simulink model "Leg_mech"  (R2015a)
settings: Solver=ode14x  StartTime=0.0  StopTime=inf  FixedStep=0.0006  RelTol=1e-3
values from neighbouring files (symbols this model uses):
  bL = 20.5    [prms.m]    (also in runFirst.m)
  bWb = 14.5    [prms.m]    (also in runFirst.m)
  bWs = 12.5    [prms.m]    (also in runFirst.m)
  C = CM + CL/n^2    (= 0.0001377500155)    [runFirst.m]
  d2 = 0    [prms.m]    (also in runFirst.m)
  J = JM + JL/n^2    (= 0.008455500031)    [runFirst.m]
  Ka = 12    [runFirst.m]
  Kb = 0.00867    [runFirst.m]
  Ke = 1    [runFirst.m]
  Km = 4.375    [runFirst.m]
  L = 0.0006    [runFirst.m]
  n = length(varargin)    [MyDynamixel.m]    (also in runFirst.m = 254)
  R = 1.4    [runFirst.m]
undefined symbols (not defined in the file or in its folder): X, Y, Z
undefined symbols (not defined in the file): L1, L2, L3, m1, m2, m3
libraries: sm_lib x20, nesl_utility x8
settings Model: Creator=340DANILOV  LastModifiedBy=340DANILOV
settings SolverCC: ZeroCrossAlgorithm=Adaptive
settings DataIOCC: SaveOutput=off  SaveTime=off
settings DiagnosticsConfigSet: SimMechanicsRigidlyBoundBlock=none

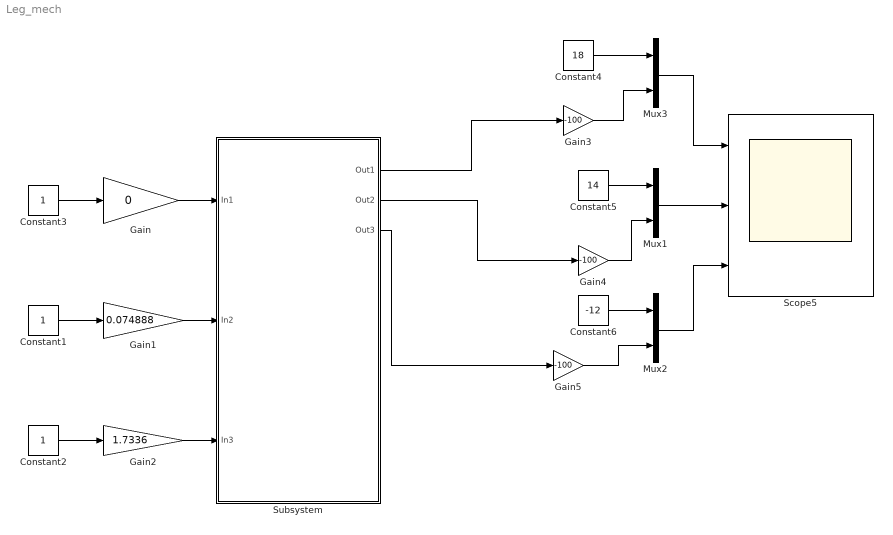
== system Leg_mech ==
  Constant1 : Constant
  Constant2 : Constant
  Constant3 : Constant
  Constant4 : Constant  Value=18
  Constant5 : Constant  Value=14
  Constant6 : Constant  Value=-12
  Gain : Gain  Gain=0
  Gain1 : Gain  Gain=0.074888
  Gain2 : Gain  Gain=1.7336
  Gain3 : Gain  Gain=-100
  Gain4 : Gain  Gain=-100
  Gain5 : Gain  Gain=-100
  Mux1 : Mux  Inputs=2
  Mux2 : Mux  Inputs=2
  Mux3 : Mux  Inputs=2
  Scope5 : Scope  NumInputPorts=3
      settings: YMin=14~14~-12.5  YMax=28~25~12.5  SaveName=ScopeData4
  Subsystem : Subsystem
  wires:
  Constant3/1 -> Gain/1
  Constant1/1 -> Gain1/1
  Constant2/1 -> Gain2/1
  Gain/1 -> Subsystem/1(In1)
  Gain1/1 -> Subsystem/2(In2)
  Gain2/1 -> Subsystem/3(In3)
  Mux2/1 -> Scope5/3
  Subsystem/1(Out1) -> Gain3/1
  Subsystem/2(Out2) -> Gain4/1
  Subsystem/3(Out3) -> Gain5/1
  Mux3/1 -> Scope5/1
  Mux1/1 -> Scope5/2
  Constant4/1 -> Mux3/1
  Gain3/1 -> Mux3/2
  Constant5/1 -> Mux1/1
  Gain4/1 -> Mux1/2
  Constant6/1 -> Mux2/1
  Gain5/1 -> Mux2/2

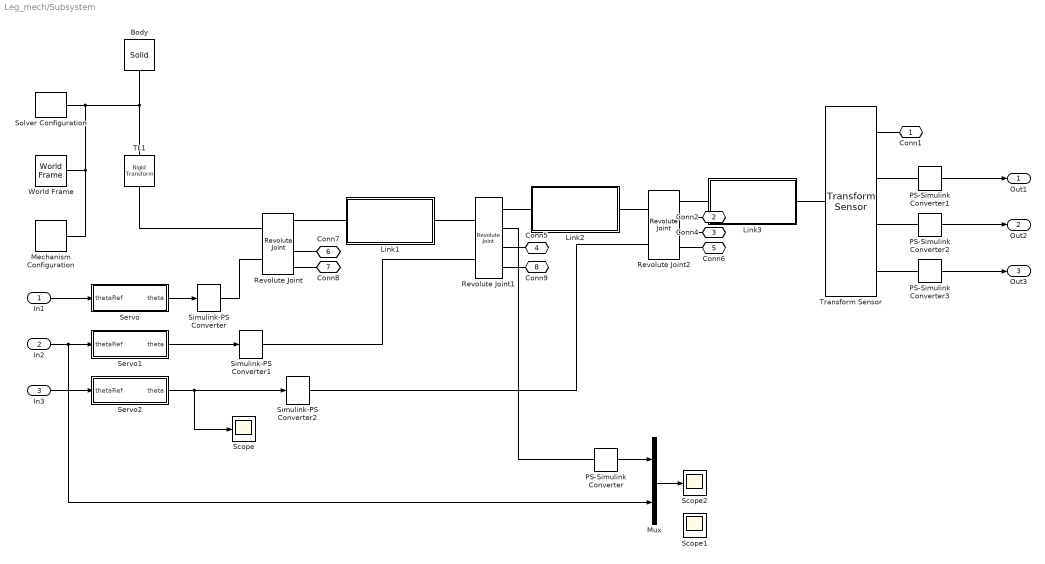
== system Leg_mech/Subsystem ==
  In1 : Inport
  In2 : Inport  Port=2
  In3 : Inport  Port=3
  Body : sm_lib/Body Elements/Solid  InertiaType=CalculateFromGeometry  Mass=0.835  MassUnits=kg  CenterOfMass=[0 0 0]  CenterOfMassUnits=m  MomentsOfInertia=[1 1 1]  MomentsOfInertiaUnits=kg*m^2  ProductsOfInertia=[0 0 0]  ProductsOfInertiaUnits=kg*m^2  DensityBased=off  Density=5000  DensityUnits=kg/(m^3)  GraphicType=FromGeometry  MarkerShape=Sphere  MarkerSize=10  MarkerSizeUnits=m  GraphicVisPropType=SimpleVisualProperties  GraphicDiffuseColor=[0.0 0.4 0.0]  GraphicSpecularColor=[0.5 0.5 0.5 1.0]  GraphicAmbientColor=[0.15 0.15 0.15 1.0]  GraphicEmissiveColor=[0.0 0.0 0.0 1.0]  GraphicShininess=75  GraphicOpacity=1.0  GeometryShape=GeneralExtrusion  RectangleSize=[1 1]  RectangleSizeUnits=m  BrickDimensions=[18.5 12.5 1]  BrickDimensionUnits=cm  CylinderRadius=1  CylinderRadiusUnits=m  CylinderLength=1  CylinderLengthUnits=m  SphereRadius=1  SphereRadiusUnits=m  EllipsoidRadii=[1 1 1]  EllipsoidRadiiUnits=m  ExtrusionCrossSection=[bL/2 bWs/2; 0 bWb/2; -bL/2 bWs/2; -bL/2 -bWs/2; 0 -bWb/2; bL/2 -bWs/2]  ExtrusionCrossSectionUnits=cm  ExtrusionLength=bH  ExtrusionLengthUnits=cm  PolygonNumSides=3  PolygonOuterRadius=1  PolygonOuterRadiusUnits=m  ExtGeomFileType=STEP  ExtGeomFileName=D:\Институт\Высертация\Model\3d\Body.STEP  ExtGeomFileUnits=m  RevolutionCrossSection=[1 1; 1 -1; 2 -1; 2 1]  RevolutionCrossSectionUnits=m  RevolutionExtent=Full  RevolutionAngle=180  RevolutionAngleUnits=deg  BlockFunction=simmechanics.library.body_elements.solid
  Link1 : Subsystem  mask{L=L1, W=1, H=1, m=m1, rgb=[0.1 0.1 0.90], Xangle=90, d1=-2.3}
      mask prompts: L "Length (cm)"; W "Width (cm)"; H "Thickness (cm)"; m "Mass (kg)"; rgb "Color [R G B]"; Xangle "+X Rotation (deg)"
      mask Display:
      | text(5,10, 'Link')
      | image(imread('sm_smpl_body.png'))
      | port_label('LConn',1,'L')
      | port_label('RConn',1,'R')
  Link2 : Subsystem  mask{L=L2, W=1, H=1, m=m2, rgb=[0.1 0.9 0.1], Xangle=180}
      mask prompts: L "Length (cm)"; W "Width (cm)"; H "Thickness (cm)"; m "Mass (kg)"; rgb "Color [R G B]"; Xangle "+X Rotation (deg)"
      mask Display:
      | text(5,10, 'Link')
      | image(imread('sm_smpl_body.png'))
      | port_label('LConn',1,'L')
      | port_label('RConn',1,'R')
  Link3 : Subsystem  mask{L=L3, W=1, H=1, m=m3, rgb=[0.9 0.1 0.10], Xangle=0}
      mask prompts: L "Length (cm)"; W "Width (cm)"; H "Thickness (cm)"; m "Mass (kg)"; rgb "Color [R G B]"; Xangle "+X Rotation (deg)"
      mask Display:
      | text(5,10, 'Link')
      | image(imread('sm_smpl_body.png'))
      | port_label('LConn',1,'L')
      | port_label('RConn',1,'R')
  Mechanism Configuration : sm_lib/Utilities/Mechanism Configuration  UniformGravity=Constant  GravityVector=[0 0 -9.80665]  GravityUnits=m/s^2  LinearizationDelta=0.001  BlockFunction=simmechanics.library.utilities.mechanism_configuration
  Mux : Mux  Inputs=2
  PS-Simulink Converter{,1..3} (4 alike) : nesl_utility/PS-Simulink Converter  PhysicalDomain=network_engine_domain  SubClassName=ps_output  LeftPortType=input  RightPortType=output  PseudoPeriodic=off  Frequencies=[]  Unit=1  AffineConversion=off
  Revolute Joint : sm_lib/Joints/Revolute Joint  SenseConstraintForce=off  SenseConstraintForceX=off  SenseConstraintForceY=off  SenseConstraintForceZ=off  SenseConstraintTorque=off  SenseConstraintTorqueX=off  SenseConstraintTorqueY=off  SenseConstraintTorqueZ=off  SenseTotalForce=off  SenseTotalForceX=off  SenseTotalForceY=off  SenseTotalForceZ=off  SenseTotalTorque=on  SenseTotalTorqueX=off  SenseTotalTorqueY=off  SenseTotalTorqueZ=off  CompositeWrenchDir=FollowerOnBase  CompositeWrenchFrame=BaseFrame  EquilibriumPosition=0  EquilibriumPositionUnits=deg  SpringStiffness=0  SpringStiffnessUnits=N*m/deg  DampingCoefficient=0  DampingCoefficientUnits=N*m/(deg/s)  TorqueActuationMode=ComputedTorque  MotionActuationMode=InputMotion  SensePosition=on  SenseVelocity=off  SenseAcceleration=off  SenseTorqueForce=on  PositionTargetSpecify=off  PositionTargetPriority=High  PositionTargetValue=0  PositionTargetValueUnits=deg  VelocityTargetSpecify=off  VelocityTargetPriority=High  VelocityTargetValue=0  VelocityTargetValueUnits=deg/s  BlockFunction=simmechanics.library.joints.revolute_joint
  Revolute Joint1 : sm_lib/Joints/Revolute Joint  SenseConstraintForce=off  SenseConstraintForceX=off  SenseConstraintForceY=off  SenseConstraintForceZ=off  SenseConstraintTorque=off  SenseConstraintTorqueX=off  SenseConstraintTorqueY=off  SenseConstraintTorqueZ=off  SenseTotalForce=off  SenseTotalForceX=off  SenseTotalForceY=off  SenseTotalForceZ=off  SenseTotalTorque=on  SenseTotalTorqueX=off  SenseTotalTorqueY=off  SenseTotalTorqueZ=off  CompositeWrenchDir=FollowerOnBase  CompositeWrenchFrame=BaseFrame  EquilibriumPosition=0  EquilibriumPositionUnits=deg  SpringStiffness=0  SpringStiffnessUnits=N*m/deg  DampingCoefficient=0  DampingCoefficientUnits=N*m/(deg/s)  TorqueActuationMode=ComputedTorque  MotionActuationMode=InputMotion  SensePosition=on  SenseVelocity=off  SenseAcceleration=off  SenseTorqueForce=on  PositionTargetSpecify=off  PositionTargetPriority=High  PositionTargetValue=0  PositionTargetValueUnits=deg  VelocityTargetSpecify=off  VelocityTargetPriority=High  VelocityTargetValue=0  VelocityTargetValueUnits=deg/s  BlockFunction=simmechanics.library.joints.revolute_joint
  Revolute Joint2 : sm_lib/Joints/Revolute Joint  SenseConstraintForce=off  SenseConstraintForceX=off  SenseConstraintForceY=off  SenseConstraintForceZ=off  SenseConstraintTorque=off  SenseConstraintTorqueX=off  SenseConstraintTorqueY=off  SenseConstraintTorqueZ=off  SenseTotalForce=off  SenseTotalForceX=off  SenseTotalForceY=off  SenseTotalForceZ=off  SenseTotalTorque=on  SenseTotalTorqueX=off  SenseTotalTorqueY=off  SenseTotalTorqueZ=off  CompositeWrenchDir=FollowerOnBase  CompositeWrenchFrame=BaseFrame  EquilibriumPosition=0  EquilibriumPositionUnits=deg  SpringStiffness=0  SpringStiffnessUnits=N*m/deg  DampingCoefficient=0  DampingCoefficientUnits=N*m/(deg/s)  TorqueActuationMode=ComputedTorque  MotionActuationMode=InputMotion  SensePosition=on  SenseVelocity=off  SenseAcceleration=off  SenseTorqueForce=on  PositionTargetSpecify=off  PositionTargetPriority=High  PositionTargetValue=0  PositionTargetValueUnits=deg  VelocityTargetSpecify=off  VelocityTargetPriority=High  VelocityTargetValue=0  VelocityTargetValueUnits=deg/s  BlockFunction=simmechanics.library.joints.revolute_joint
  Scope : Scope
  Scope1 : Scope
  Scope2 : Scope
      settings: YMin=0.025  YMax=0.3  SaveName=ScopeData2
  Servo : Subsystem
  Servo1 : Subsystem
  Servo2 : Subsystem
  Simulink-PS Converter : nesl_utility/Simulink-PS Converter  PhysicalDomain=network_engine_domain  SubClassName=ps_input  LeftPortType=input  RightPortType=output  PseudoPeriodic=off  Frequencies=[]  NoiseDistribution=none  NoiseParameters=[]  Unit=1  AffineConversion=off  InputFiltering=on  SimscapeFilterOrder=2  InputFilterTimeConstant=0.001  UdotUserProvided=1
  Simulink-PS Converter1 : nesl_utility/Simulink-PS Converter  PhysicalDomain=network_engine_domain  SubClassName=ps_input  LeftPortType=input  RightPortType=output  PseudoPeriodic=off  Frequencies=[]  NoiseDistribution=none  NoiseParameters=[]  Unit=1  AffineConversion=off  InputFiltering=on  SimscapeFilterOrder=2  InputFilterTimeConstant=0.001  UdotUserProvided=1
  Simulink-PS Converter2 : nesl_utility/Simulink-PS Converter  PhysicalDomain=network_engine_domain  SubClassName=ps_input  LeftPortType=input  RightPortType=output  PseudoPeriodic=off  Frequencies=[]  NoiseDistribution=none  NoiseParameters=[]  Unit=1  AffineConversion=off  InputFiltering=on  SimscapeFilterOrder=2  InputFilterTimeConstant=0.001  UdotUserProvided=1
  Solver Configuration : nesl_utility/Solver Configuration  PhysicalDomain=network_engine_domain  SubClassName=solver  LeftPortType=input  RightPortType=generic  Accelerate=off  Tones=[]  Harmonics=[]  SimulateNoise=off  Profile=off  UseLocalSampling=off  EnableSwitchedLinearOptims=on  FrequencyDomain=off  UseCCode=off  RelTol=0.001  AbsTol=1e-06  MinStep=1e-09  ToWorkspace=off  RevertToSquareIcSolve=off  NumHomotopyIterations=100  DoDC=off  ResidualTolerance=1e-09  UseLocalSolver=off  LocalSolverChoice=NE_BACKWARD_EULER_ADVANCER  LocalSolverSampleTime=0.001  DoFixedCost=off  MaxNonlinIter=3  MaxModeIter=2  LinearAlgebra=Sparse  DelaysMemoryBudget=1024  AutomaticFiltering=on  FilteringTimeConstant=0.001
  TL1 : sm_lib/Frames and Transforms/Rigid Transform  TranslationMethod=Cartesian  TranslationLengthUnit=cm  TranslationStandardAxis=+Z  TranslationStandardOffset=0  TranslationCartesianOffset=[bL/2 bWs/2 0]  TranslationROffset=0  TranslationROffsetUnits=m  TranslationZOffset=0  TranslationZOffsetUnits=m  TranslationThetaOffset=0  TranslationThetaOffsetUnits=deg  RotationMethod=StandardAxis  RotationAngleUnits=deg  RotationStandardAxis=+Z  RotationAngle=90-45  RotationArbitraryAxis=[0 0 1]  FollAlignAxisA=+X  BaseAlignAxisA=+Y  FollAlignAxisB=+Y  BaseAlignAxisB=+Z  RotationMatrix=[1 0 0; 0 1 0; 0 0 1]  BlockFunction=simmechanics.library.frames_transforms.rigid_transform
  Transform Sensor : sm_lib/Frames and Transforms/Transform Sensor  MeasurementFrame=World  SenseAngle=off  SenseAxis=off  SenseAngle1=off  SenseAngle2=off  SenseAngle3=off  SenseQ=off  SenseR=off  SenseOmegaX=off  SenseOmegaY=off  SenseOmegaZ=off  SenseOmega1=off  SenseOmega2=off  SenseOmega3=off  SenseQDot=off  SenseRDot=off  SenseAlphaX=off  SenseAlphaY=off  SenseAlphaZ=off  SenseAlpha1=off  SenseAlpha2=off  SenseAlpha3=off  SenseQDDot=off  SenseRDDot=off  SenseX=on  SenseY=on  SenseZ=on  SenseRad=off  SenseAzim=off  SenseDist=off  SenseInc=off  SenseXDot=off  SenseYDot=off  SenseZDot=off  SenseRadDot=off  SenseAzimDot=off  SenseDistDot=off  SenseIncDot=off  SenseXDDot=off  SenseYDDot=off  SenseZDDot=off  SenseRadDDot=off  SenseAzimDDot=off  SenseDistDDot=off  SenseIncDDot=off  BlockFunction=simmechanics.library.frames_transforms.transform_sensor
  World Frame : sm_lib/Frames and Transforms/World Frame  BlockFunction=simmechanics.library.frames_transforms.world_frame
  Conn1 : PMIOPort  Port=1  Side=Right
  Conn2 : PMIOPort  Port=2  Side=Right
  Conn4 : PMIOPort  Port=3  Side=Right
  Conn5 : PMIOPort  Port=4  Side=Right
  Conn6 : PMIOPort  Port=5  Side=Right
  Conn7 : PMIOPort  Port=6  Side=Right
  Conn8 : PMIOPort  Port=7  Side=Right
  Conn9 : PMIOPort  Port=8  Side=Right
  Out1 : Outport
  Out2 : Outport  Port=2
  Out3 : Outport  Port=3
  wires:
  PS-Simulink Converter2/1 -> Out2/1
  PS-Simulink Converter1/1 -> Out1/1
  Servo/1(theta) -> Simulink-PS Converter/1
  Servo2/1(theta) -> Scope/1, Simulink-PS Converter2/1
  Servo1/1(theta) -> Simulink-PS Converter1/1
  In1/1 -> Servo/1(thetaRef)
  In2/1 -> Mux/2, Servo1/1(thetaRef)
  In3/1 -> Servo2/1(thetaRef)
  PS-Simulink Converter3/1 -> Out3/1
  PS-Simulink Converter/1 -> Mux/1
  Mux/1 -> Scope2/1
  connections:
  PS-Simulink Converter1/LConn1 -- Transform Sensor/RConn2
  World Frame/RConn1 -- Mechanism Configuration/RConn1 -- Body/RConn1 -- TL1/LConn1 -- Solver Configuration/RConn1
  Revolute Joint/LConn1 -- TL1/RConn1
  Link1/LConn1 -- Revolute Joint/RConn1
  Revolute Joint1/LConn1 -- Link1/RConn1
  Link2/LConn1 -- Revolute Joint1/RConn1
  Revolute Joint2/LConn1 -- Link2/RConn1
  Link3/LConn1 -- Revolute Joint2/RConn1
  Revolute Joint/LConn2 -- Simulink-PS Converter/RConn1
  Simulink-PS Converter1/RConn1 -- Revolute Joint1/LConn2
  Simulink-PS Converter2/RConn1 -- Revolute Joint2/LConn2
  Transform Sensor/RConn1 -- Conn1/RConn1
  Revolute Joint/RConn4 -- Conn8/RConn1
  Revolute Joint1/RConn3 -- Conn5/RConn1
  Revolute Joint1/RConn4 -- Conn9/RConn1
  Revolute Joint2/RConn4 -- Conn6/RConn1
  Revolute Joint2/RConn3 -- Conn4/RConn1
  PS-Simulink Converter/LConn1 -- Revolute Joint1/RConn2
  Revolute Joint2/RConn2 -- Conn2/RConn1
  Revolute Joint/RConn3 -- Conn7/RConn1
  PS-Simulink Converter2/LConn1 -- Transform Sensor/RConn3
  Transform Sensor/LConn1 -- Link3/RConn1
  PS-Simulink Converter3/LConn1 -- Transform Sensor/RConn4

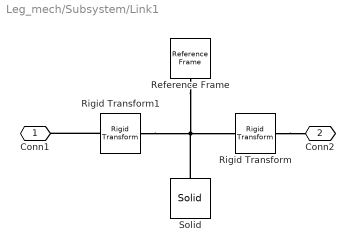
== system Leg_mech/Subsystem/Link1 ==
  Reference Frame : sm_lib/Frames and Transforms/Reference Frame  BlockFunction=simmechanics.library.frames_transforms.reference_frame
  Rigid Transform : sm_lib/Frames and Transforms/Rigid Transform  TranslationMethod=Cartesian  TranslationLengthUnit=cm  TranslationStandardAxis=+X  TranslationStandardOffset=L/2  TranslationCartesianOffset=[L/2 0 d2]  TranslationROffset=0  TranslationROffsetUnits=m  TranslationZOffset=0  TranslationZOffsetUnits=m  TranslationThetaOffset=0  TranslationThetaOffsetUnits=deg  RotationMethod=StandardAxis  RotationAngleUnits=deg  RotationStandardAxis=+X  RotationAngle=Xangle  RotationArbitraryAxis=[0 0 1]  FollAlignAxisA=+X  BaseAlignAxisA=+Y  FollAlignAxisB=+Y  BaseAlignAxisB=+Z  RotationMatrix=[1 0 0; 0 1 0; 0 0 1]  BlockFunction=simmechanics.library.frames_transforms.rigid_transform
  Rigid Transform1 : sm_lib/Frames and Transforms/Rigid Transform  TranslationMethod=StandardAxis  TranslationLengthUnit=cm  TranslationStandardAxis=-X  TranslationStandardOffset=L/2  TranslationCartesianOffset=[0 0 0]  TranslationROffset=0  TranslationROffsetUnits=m  TranslationZOffset=0  TranslationZOffsetUnits=m  TranslationThetaOffset=0  TranslationThetaOffsetUnits=deg  RotationMethod=None  RotationAngleUnits=deg  RotationStandardAxis=+Z  RotationAngle=0.0  RotationArbitraryAxis=[0 0 1]  FollAlignAxisA=+X  BaseAlignAxisA=+Y  FollAlignAxisB=+Y  BaseAlignAxisB=+Z  RotationMatrix=[1 0 0; 0 1 0; 0 0 1]  BlockFunction=simmechanics.library.frames_transforms.rigid_transform
  Solid : sm_lib/Body Elements/Solid  InertiaType=PointMass  Mass=m  MassUnits=kg  CenterOfMass=[0 0 0]  CenterOfMassUnits=m  MomentsOfInertia=[1 1 1]  MomentsOfInertiaUnits=kg*m^2  ProductsOfInertia=[0 0 0]  ProductsOfInertiaUnits=kg*m^2  DensityBased=off  Density=1  DensityUnits=kg/(m^3)  GraphicType=FromGeometry  MarkerShape=Sphere  MarkerSize=10  MarkerSizeUnits=m  GraphicVisPropType=SimpleVisualProperties  GraphicDiffuseColor=rgb  GraphicSpecularColor=[0.5 0.5 0.5 1.0]  GraphicAmbientColor=[0.15 0.15 0.15 1.0]  GraphicEmissiveColor=[0.0 0.0 0.0 1.0]  GraphicShininess=75  GraphicOpacity=1.0  GeometryShape=Brick  RectangleSize=[1 1]  RectangleSizeUnits=m  BrickDimensions=[L 1 1]  BrickDimensionUnits=cm  CylinderRadius=1  CylinderRadiusUnits=m  CylinderLength=1  CylinderLengthUnits=m  SphereRadius=1  SphereRadiusUnits=m  EllipsoidRadii=[1 1 1]  EllipsoidRadiiUnits=m  ExtrusionCrossSection=[1 1; -1 1; -1 -1; 1 -1]  ExtrusionCrossSectionUnits=m  ExtrusionLength=1  ExtrusionLengthUnits=m  PolygonNumSides=3  PolygonOuterRadius=1  PolygonOuterRadiusUnits=m  ExtGeomFileType=STEP  ExtGeomFileName=D:\Институт\Высертация\Model\3d\Link1.STEP  ExtGeomFileUnits=m  RevolutionCrossSection=[1 1; 1 -1; 2 -1; 2 1]  RevolutionCrossSectionUnits=m  RevolutionExtent=Full  RevolutionAngle=180  RevolutionAngleUnits=deg  BlockFunction=simmechanics.library.body_elements.solid
  Conn1 : PMIOPort  Port=1  Side=Left
  Conn2 : PMIOPort  Port=2  Side=Right
  connections:
  Reference Frame/RConn1 -- Solid/RConn1 -- Rigid Transform/LConn1 -- Rigid Transform1/LConn1
  Rigid Transform/RConn1 -- Conn2/RConn1
  Rigid Transform1/RConn1 -- Conn1/RConn1

== system Leg_mech/Subsystem/Link2 ==
  Reference Frame : sm_lib/Frames and Transforms/Reference Frame  BlockFunction=simmechanics.library.frames_transforms.reference_frame
  Rigid Transform : sm_lib/Frames and Transforms/Rigid Transform  TranslationMethod=StandardAxis  TranslationLengthUnit=cm  TranslationStandardAxis=+X  TranslationStandardOffset=L/2  TranslationCartesianOffset=[0 0 0]  TranslationROffset=0  TranslationROffsetUnits=m  TranslationZOffset=0  TranslationZOffsetUnits=m  TranslationThetaOffset=0  TranslationThetaOffsetUnits=deg  RotationMethod=StandardAxis  RotationAngleUnits=deg  RotationStandardAxis=+X  RotationAngle=Xangle  RotationArbitraryAxis=[0 0 1]  FollAlignAxisA=+X  BaseAlignAxisA=+Y  FollAlignAxisB=+Y  BaseAlignAxisB=+Z  RotationMatrix=[1 0 0; 0 1 0; 0 0 1]  BlockFunction=simmechanics.library.frames_transforms.rigid_transform
  Rigid Transform1 : sm_lib/Frames and Transforms/Rigid Transform  TranslationMethod=StandardAxis  TranslationLengthUnit=cm  TranslationStandardAxis=-X  TranslationStandardOffset=L/2  TranslationCartesianOffset=[0 0 0]  TranslationROffset=0  TranslationROffsetUnits=m  TranslationZOffset=0  TranslationZOffsetUnits=m  TranslationThetaOffset=0  TranslationThetaOffsetUnits=deg  RotationMethod=None  RotationAngleUnits=deg  RotationStandardAxis=+Z  RotationAngle=0.0  RotationArbitraryAxis=[0 0 1]  FollAlignAxisA=+X  BaseAlignAxisA=+Y  FollAlignAxisB=+Y  BaseAlignAxisB=+Z  RotationMatrix=[1 0 0; 0 1 0; 0 0 1]  BlockFunction=simmechanics.library.frames_transforms.rigid_transform
  Solid : sm_lib/Body Elements/Solid  InertiaType=PointMass  Mass=m  MassUnits=kg  CenterOfMass=[0 0 0]  CenterOfMassUnits=m  MomentsOfInertia=[1 1 1]  MomentsOfInertiaUnits=kg*m^2  ProductsOfInertia=[0 0 0]  ProductsOfInertiaUnits=kg*m^2  DensityBased=off  Density=1  DensityUnits=kg/(m^3)  GraphicType=FromGeometry  MarkerShape=Sphere  MarkerSize=10  MarkerSizeUnits=m  GraphicVisPropType=SimpleVisualProperties  GraphicDiffuseColor=rgb  GraphicSpecularColor=[0.5 0.5 0.5 1.0]  GraphicAmbientColor=[0.15 0.15 0.15 1.0]  GraphicEmissiveColor=[0.0 0.0 0.0 1.0]  GraphicShininess=75  GraphicOpacity=1.0  GeometryShape=Brick  RectangleSize=[1 1]  RectangleSizeUnits=m  BrickDimensions=[L W H]  BrickDimensionUnits=cm  CylinderRadius=1  CylinderRadiusUnits=m  CylinderLength=1  CylinderLengthUnits=m  SphereRadius=1  SphereRadiusUnits=m  EllipsoidRadii=[1 1 1]  EllipsoidRadiiUnits=m  ExtrusionCrossSection=[1 1; -1 1; -1 -1; 1 -1]  ExtrusionCrossSectionUnits=m  ExtrusionLength=1  ExtrusionLengthUnits=m  PolygonNumSides=3  PolygonOuterRadius=1  PolygonOuterRadiusUnits=m  ExtGeomFileType=STEP  ExtGeomFileName=D:\Институт\Высертация\Model\3d\Link2.STEP  ExtGeomFileUnits=m  RevolutionCrossSection=[1 1; 1 -1; 2 -1; 2 1]  RevolutionCrossSectionUnits=m  RevolutionExtent=Full  RevolutionAngle=180  RevolutionAngleUnits=deg  BlockFunction=simmechanics.library.body_elements.solid
  Conn1 : PMIOPort  Port=1  Side=Left
  Conn2 : PMIOPort  Port=2  Side=Right
  connections:
  Rigid Transform1/RConn1 -- Conn1/RConn1
  Rigid Transform/RConn1 -- Conn2/RConn1
  Rigid Transform1/LConn1 -- Rigid Transform/LConn1 -- Solid/RConn1 -- Reference Frame/RConn1

== system Leg_mech/Subsystem/Link3 ==
  Reference Frame : sm_lib/Frames and Transforms/Reference Frame  BlockFunction=simmechanics.library.frames_transforms.reference_frame
  Rigid Transform : sm_lib/Frames and Transforms/Rigid Transform  TranslationMethod=StandardAxis  TranslationLengthUnit=cm  TranslationStandardAxis=+X  TranslationStandardOffset=L/2  TranslationCartesianOffset=[0 0 0]  TranslationROffset=0  TranslationROffsetUnits=m  TranslationZOffset=0  TranslationZOffsetUnits=m  TranslationThetaOffset=0  TranslationThetaOffsetUnits=deg  RotationMethod=None  RotationAngleUnits=deg  RotationStandardAxis=+X  RotationAngle=Xangle  RotationArbitraryAxis=[0 0 1]  FollAlignAxisA=+X  BaseAlignAxisA=+Y  FollAlignAxisB=+Y  BaseAlignAxisB=+Z  RotationMatrix=[1 0 0; 0 1 0; 0 0 1]  BlockFunction=simmechanics.library.frames_transforms.rigid_transform
  Rigid Transform1 : sm_lib/Frames and Transforms/Rigid Transform  TranslationMethod=StandardAxis  TranslationLengthUnit=cm  TranslationStandardAxis=-X  TranslationStandardOffset=L/2  TranslationCartesianOffset=[0 0 0]  TranslationROffset=0  TranslationROffsetUnits=m  TranslationZOffset=0  TranslationZOffsetUnits=m  TranslationThetaOffset=0  TranslationThetaOffsetUnits=deg  RotationMethod=None  RotationAngleUnits=deg  RotationStandardAxis=+Z  RotationAngle=0.0  RotationArbitraryAxis=[0 0 1]  FollAlignAxisA=+X  BaseAlignAxisA=+Y  FollAlignAxisB=+Y  BaseAlignAxisB=+Z  RotationMatrix=[1 0 0; 0 1 0; 0 0 1]  BlockFunction=simmechanics.library.frames_transforms.rigid_transform
  Solid : sm_lib/Body Elements/Solid  InertiaType=PointMass  Mass=m  MassUnits=kg  CenterOfMass=[0 0 0]  CenterOfMassUnits=m  MomentsOfInertia=[1 1 1]  MomentsOfInertiaUnits=kg*m^2  ProductsOfInertia=[0 0 0]  ProductsOfInertiaUnits=kg*m^2  DensityBased=off  Density=1  DensityUnits=kg/(m^3)  GraphicType=FromGeometry  MarkerShape=Sphere  MarkerSize=10  MarkerSizeUnits=m  GraphicVisPropType=SimpleVisualProperties  GraphicDiffuseColor=rgb  GraphicSpecularColor=[0.5 0.5 0.5 1.0]  GraphicAmbientColor=[0.15 0.15 0.15 1.0]  GraphicEmissiveColor=[0.0 0.0 0.0 1.0]  GraphicShininess=75  GraphicOpacity=1.0  GeometryShape=Brick  RectangleSize=[1 1]  RectangleSizeUnits=m  BrickDimensions=[L W H]  BrickDimensionUnits=cm  CylinderRadius=1  CylinderRadiusUnits=m  CylinderLength=1  CylinderLengthUnits=m  SphereRadius=1  SphereRadiusUnits=m  EllipsoidRadii=[1 1 1]  EllipsoidRadiiUnits=m  ExtrusionCrossSection=[1 1; -1 1; -1 -1; 1 -1]  ExtrusionCrossSectionUnits=m  ExtrusionLength=1  ExtrusionLengthUnits=m  PolygonNumSides=3  PolygonOuterRadius=1  PolygonOuterRadiusUnits=m  ExtGeomFileType=STEP  ExtGeomFileName=D:\Институт\Высертация\Model\3d\link3.STEP  ExtGeomFileUnits=m  RevolutionCrossSection=[1 1; 1 -1; 2 -1; 2 1]  RevolutionCrossSectionUnits=m  RevolutionExtent=Full  RevolutionAngle=180  RevolutionAngleUnits=deg  BlockFunction=simmechanics.library.body_elements.solid
  Conn1 : PMIOPort  Port=1  Side=Left
  Conn2 : PMIOPort  Port=2  Side=Right
  connections:
  Reference Frame/RConn1 -- Solid/RConn1 -- Rigid Transform/LConn1 -- Rigid Transform1/LConn1
  Rigid Transform/RConn1 -- Conn2/RConn1
  Rigid Transform1/RConn1 -- Conn1/RConn1

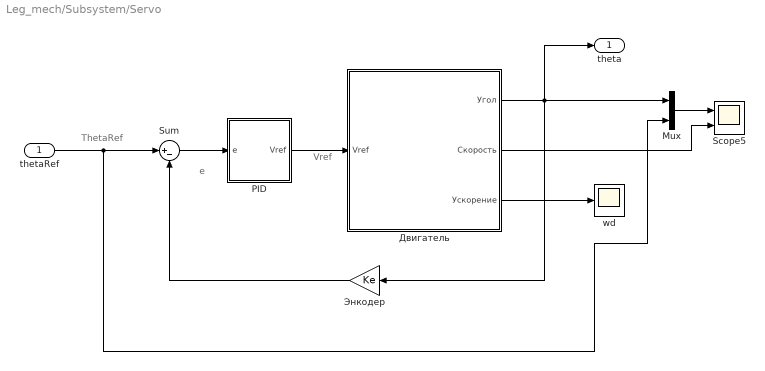
== system Leg_mech/Subsystem/Servo ==
  note: ThetaRef
  note: e
  note: Vref
  thetaRef : Inport
  Mux : Mux  Inputs=2
  PID : Subsystem
  Scope5 : Scope  NumInputPorts=2
      settings: YMin=5.55112e-17~-3.5  YMax=1.1~3.5  SaveName=ScopeData45
  Sum : Sum  Inputs=|+-
  wd : Scope
      settings: SaveName=ScopeData3
  Двигатель : Subsystem
  Энкодер : Gain  Gain=Ke
  theta : Outport
  wires:
  Mux/1 -> Scope5/1
  Двигатель/3(Ускорение) -> wd/1
  PID/1(Vref) -> Двигатель/1(Vref)
  Двигатель/1(Угол) -> Энкодер/1, theta/1, Mux/1
  Энкодер/1 -> Sum/2
  Sum/1 -> PID/1(e)
  thetaRef/1 -> Sum/1, Mux/2
  Двигатель/2(Скорость) -> Scope5/2

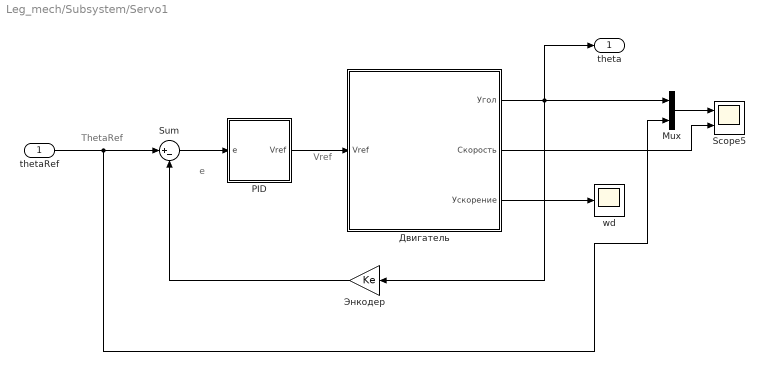
== system Leg_mech/Subsystem/Servo1 ==
  note: ThetaRef
  note: e
  note: Vref
  thetaRef : Inport
  Mux : Mux  Inputs=2
  PID : Subsystem
  Scope5 : Scope  NumInputPorts=2
      settings: YMin=-0.28285~-0.0045  YMax=-0.2824~0  SaveName=ScopeData45
  Sum : Sum  Inputs=|+-
  wd : Scope
      settings: SaveName=ScopeData3
  Двигатель : Subsystem
  Энкодер : Gain  Gain=Ke
  theta : Outport
  wires:
  Mux/1 -> Scope5/1
  Двигатель/3(Ускорение) -> wd/1
  PID/1(Vref) -> Двигатель/1(Vref)
  Двигатель/1(Угол) -> Энкодер/1, theta/1, Mux/1
  Энкодер/1 -> Sum/2
  Sum/1 -> PID/1(e)
  thetaRef/1 -> Sum/1, Mux/2
  Двигатель/2(Скорость) -> Scope5/2

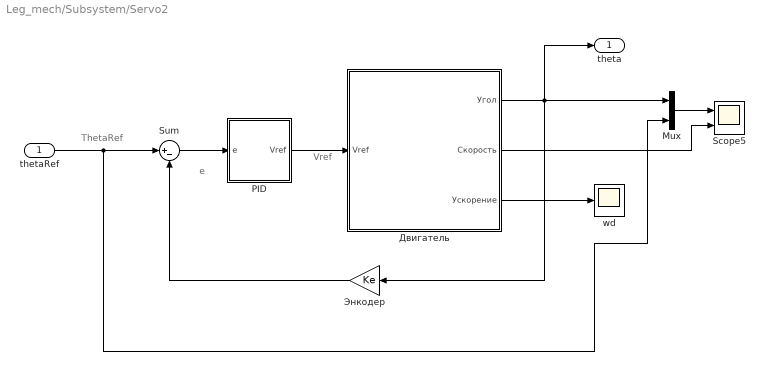
== system Leg_mech/Subsystem/Servo2 ==
  note: Vref
  note: e
  note: ThetaRef
  thetaRef : Inport
  Mux : Mux  Inputs=2
  PID : Subsystem
  Scope5 : Scope  NumInputPorts=2
      settings: YMin=1.4~-0.25  YMax=2.2~3.25  SaveName=ScopeData45
  Sum : Sum  Inputs=|+-
  wd : Scope
      settings: SaveName=ScopeData3
  Двигатель : Subsystem
  Энкодер : Gain  Gain=Ke
  theta : Outport
  wires:
  Двигатель/2(Скорость) -> Scope5/2
  thetaRef/1 -> Mux/2, Sum/1
  Sum/1 -> PID/1(e)
  Энкодер/1 -> Sum/2
  Двигатель/1(Угол) -> Mux/1, theta/1, Энкодер/1
  PID/1(Vref) -> Двигатель/1(Vref)
  Двигатель/3(Ускорение) -> wd/1
  Mux/1 -> Scope5/1

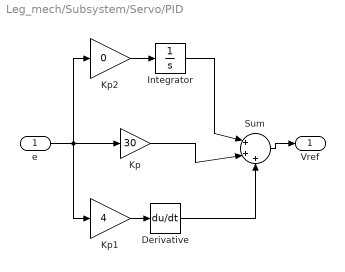
== system Leg_mech/Subsystem/Servo/PID ==
  e : Inport
  Derivative : Derivative
  Integrator : Integrator
  Kp : Gain  Gain=30
  Kp1 : Gain  Gain=4
  Kp2 : Gain  Gain=0
  Sum : Sum  Inputs=|+++
  Vref : Outport
  wires:
  Derivative/1 -> Sum/3
  Kp/1 -> Sum/2
  Integrator/1 -> Sum/1
  Kp2/1 -> Integrator/1
  Sum/1 -> Vref/1
  Kp1/1 -> Derivative/1
  e/1 -> Kp/1, Kp1/1, Kp2/1

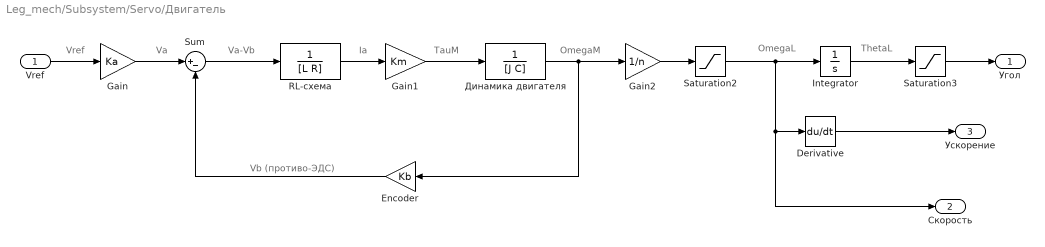
== system Leg_mech/Subsystem/Servo/Двигатель ==
  note: Vref
  note: Va
  note: Va-Vb
  note: Vb (противо-ЭДС)
  note: Ia
  note: TauM
  note: OmegaM
  note: OmegaL
  note: ThetaL
  Vref : Inport
  Derivative : Derivative
  Encoder : Gain  Gain=Kb
  Gain : Gain  Gain=Ka
  Gain1 : Gain  Gain=Km
  Gain2 : Gain  Gain=1/n
  Integrator : Integrator
  RL-схема : TransferFcn  Denominator=[L R]
  Saturation2 : Saturate  UpperLimit=190*pi/180  LowerLimit=-190*pi/180  OutMin=[-190*pi/180]  OutMax=[190*pi/180]
  Saturation3 : Saturate  UpperLimit=60*pi/180  LowerLimit=-60*pi/180  OutMin=[-150*pi/180]  OutMax=[150*pi/180]
  Sum : Sum  Inputs=|+-
  Динамика двигателя : TransferFcn  Denominator=[J C]
  Угол : Outport
  Скорость : Outport  Port=2
  Ускорение : Outport  Port=3
  wires:
  Saturation3/1 -> Угол/1
  Gain/1 -> Sum/1
  Vref/1 -> Gain/1
  Integrator/1 -> Saturation3/1
  Encoder/1 -> Sum/2
  Gain1/1 -> Динамика двигателя/1
  Sum/1 -> RL-схема/1
  RL-схема/1 -> Gain1/1
  Derivative/1 -> Ускорение/1
  Динамика двигателя/1 -> Gain2/1, Encoder/1
  Gain2/1 -> Saturation2/1
  Saturation2/1 -> Integrator/1, Скорость/1, Derivative/1

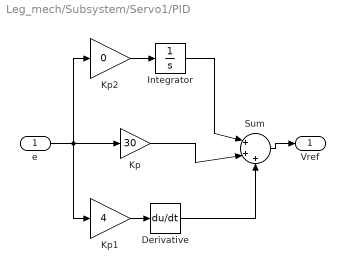
== system Leg_mech/Subsystem/Servo1/PID ==
  e : Inport
  Derivative : Derivative
  Integrator : Integrator
  Kp : Gain  Gain=30
  Kp1 : Gain  Gain=4
  Kp2 : Gain  Gain=0
  Sum : Sum  Inputs=|+++
  Vref : Outport
  wires:
  Derivative/1 -> Sum/3
  Kp/1 -> Sum/2
  Integrator/1 -> Sum/1
  Kp2/1 -> Integrator/1
  Sum/1 -> Vref/1
  Kp1/1 -> Derivative/1
  e/1 -> Kp/1, Kp1/1, Kp2/1

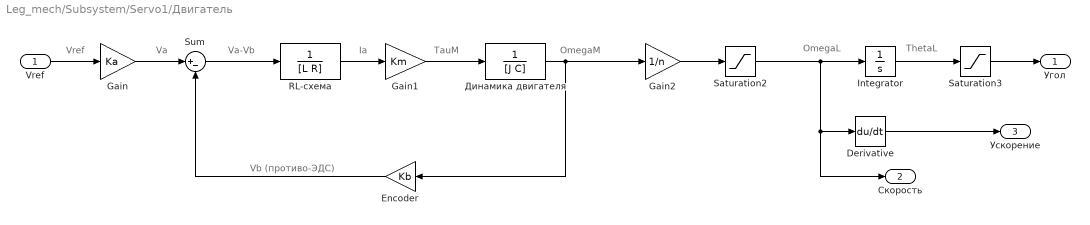
== system Leg_mech/Subsystem/Servo1/Двигатель ==
  note: Vref
  note: Va
  note: Va-Vb
  note: Vb (противо-ЭДС)
  note: Ia
  note: TauM
  note: OmegaM
  note: OmegaL
  note: ThetaL
  Vref : Inport
  Derivative : Derivative
  Encoder : Gain  Gain=Kb
  Gain : Gain  Gain=Ka
  Gain1 : Gain  Gain=Km
  Gain2 : Gain  Gain=1/n
  Integrator : Integrator
  RL-схема : TransferFcn  Denominator=[L R]
  Saturation2 : Saturate  UpperLimit=190*pi/180  LowerLimit=-190*pi/180  OutMin=[-190*pi/180]  OutMax=[190*pi/180]
  Saturation3 : Saturate  UpperLimit=90*pi/180  LowerLimit=-90*pi/180  OutMin=[-150*pi/180]  OutMax=[150*pi/180]
  Sum : Sum  Inputs=|+-
  Динамика двигателя : TransferFcn  Denominator=[J C]
  Угол : Outport
  Скорость : Outport  Port=2
  Ускорение : Outport  Port=3
  wires:
  Saturation3/1 -> Угол/1
  Gain/1 -> Sum/1
  Gain2/1 -> Saturation2/1
  Vref/1 -> Gain/1
  Integrator/1 -> Saturation3/1
  Encoder/1 -> Sum/2
  Gain1/1 -> Динамика двигателя/1
  Sum/1 -> RL-схема/1
  RL-схема/1 -> Gain1/1
  Derivative/1 -> Ускорение/1
  Динамика двигателя/1 -> Gain2/1, Encoder/1
  Saturation2/1 -> Integrator/1, Скорость/1, Derivative/1

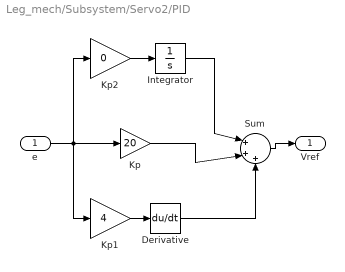
== system Leg_mech/Subsystem/Servo2/PID ==
  e : Inport
  Derivative : Derivative
  Integrator : Integrator
  Kp : Gain  Gain=20
  Kp1 : Gain  Gain=4
  Kp2 : Gain  Gain=0
  Sum : Sum  Inputs=|+++
  Vref : Outport
  wires:
  e/1 -> Kp2/1, Kp1/1, Kp/1
  Kp1/1 -> Derivative/1
  Sum/1 -> Vref/1
  Kp2/1 -> Integrator/1
  Integrator/1 -> Sum/1
  Kp/1 -> Sum/2
  Derivative/1 -> Sum/3

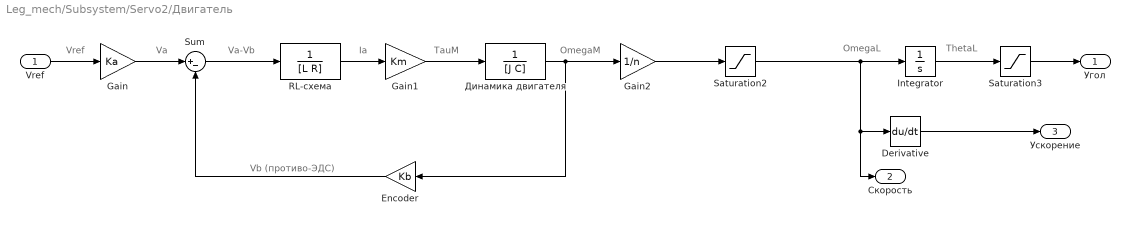
== system Leg_mech/Subsystem/Servo2/Двигатель ==
  note: ThetaL
  note: OmegaL
  note: OmegaM
  note: TauM
  note: Ia
  note: Vb (противо-ЭДС)
  note: Va-Vb
  note: Va
  note: Vref
  Vref : Inport
  Derivative : Derivative
  Encoder : Gain  Gain=Kb
  Gain : Gain  Gain=Ka
  Gain1 : Gain  Gain=Km
  Gain2 : Gain  Gain=1/n
  Integrator : Integrator
  RL-схема : TransferFcn  Denominator=[L R]
  Saturation2 : Saturate  UpperLimit=190*pi/180  LowerLimit=-190*pi/180  OutMin=[-190*pi/180]  OutMax=[190*pi/180]
  Saturation3 : Saturate  UpperLimit=150*pi/180  LowerLimit=-150*pi/180  OutMin=[-150*pi/180]  OutMax=[150*pi/180]
  Sum : Sum  Inputs=|+-
  Динамика двигателя : TransferFcn  Denominator=[J C]
  Угол : Outport
  Скорость : Outport  Port=2
  Ускорение : Outport  Port=3
  wires:
  RL-схема/1 -> Gain1/1
  Sum/1 -> RL-схема/1
  Gain1/1 -> Динамика двигателя/1
  Encoder/1 -> Sum/2
  Динамика двигателя/1 -> Gain2/1, Encoder/1
  Integrator/1 -> Saturation3/1
  Vref/1 -> Gain/1
  Gain/1 -> Sum/1
  Saturation3/1 -> Угол/1
  Derivative/1 -> Ускорение/1
  Gain2/1 -> Saturation2/1
  Saturation2/1 -> Derivative/1, Скорость/1, Integrator/1
